simulink model "control_model_flight"  (R2025b)
settings: Solver=VariableStepAuto  StartTime=0.0  StopTime=100  RelTol=1e-3
undefined symbols (not defined in the file): Am, B, Bm, Cm, Dm, engine_gimbal_speed, engine_max_angle, gain, Iy, kd, kp, Kr, Kx, P, static_margin, thrust
libraries: simulink_extras x6, simulink x2
settings Model: Creator=marti  LastModifiedBy=marti
settings DebuggingCC: AlgebraicLoopMsg=none

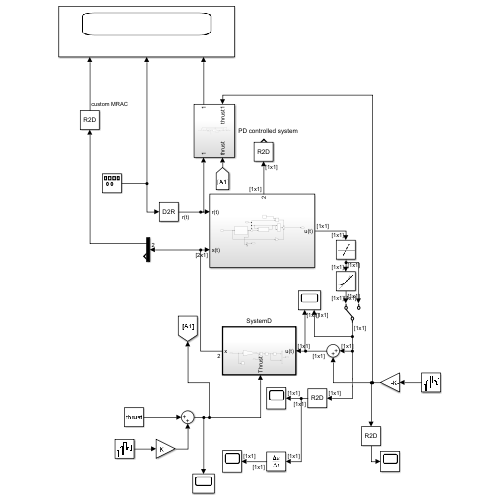
[thumbnail: Simulink's stored preview of the top-level diagram]
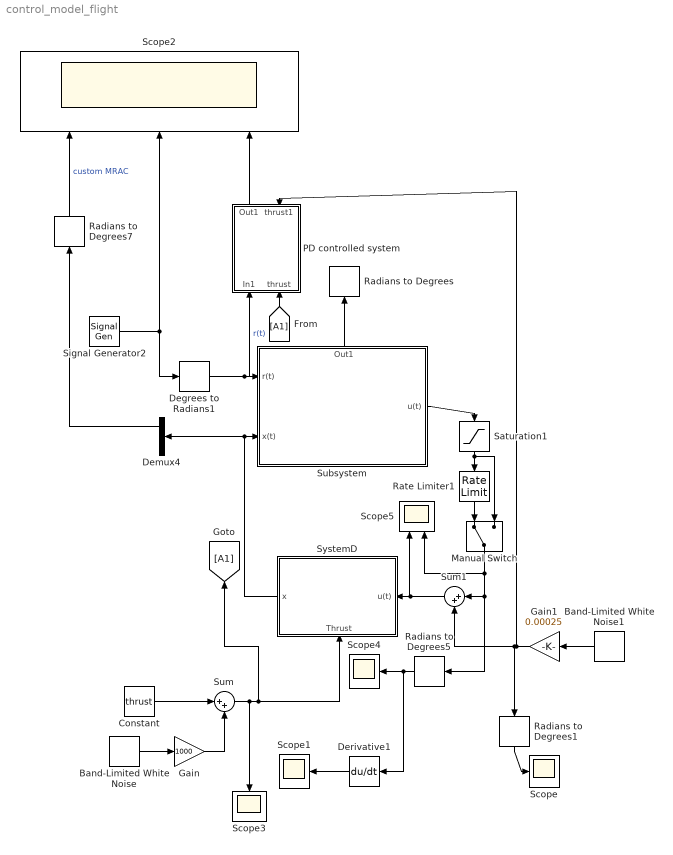
== system control_model_flight ==
  Band-Limited White Noise : simulink/Sources/Band-Limited White Noise  Cov=[0.1]  Ts=1  seed=[23341]
  Band-Limited White Noise1 : simulink/Sources/Band-Limited White Noise  Cov=[0.1]  Ts=0.001  seed=[23341]
  Constant : Constant  Value=thrust
  Degrees to Radians1 : simulink_extras/Transformations/Degrees to Radians
  Demux4 : Demux  Outputs=2
  Derivative1 : Derivative
  Gain : Gain  Gain=1000
  Gain1 : Gain  Gain=0.00025
  Manual Switch : ManualSwitch
  PD controlled system : Subsystem
      settings: PortSchema="{\"entries\":[{\"content\":{\"sides\":[{\"content\":{\"connectorIds\":[\"In1\",\"In2\"]},\"type\":\"ConnectorPlacement.EquallySpacedRectSide\",\"uuid\":\"7664c1e6-ae69-4202-b6ee-140830191e3f\"},{\"content\":{\"connectorIds\":[\"Out1\",\"In3\"],\"side\":\"RIGHT\"},\"type\":\"ConnectorPlacement.EquallySpacedRectSide\",\"uuid\":\"1121b3c6-b64f-4e76-a835-89366e6f1ec3\"},{\"content\":{\"side\":\"TOP\"},\"type\":\"ConnectorPlacement.EquallySpacedRectSide\",\"uuid\":\"4ddc513e-e9d6-44c8-bfb2-5693fffff535\"}]},\"type\":\"ConnectorPlacement.EquallySpacedConnector\",\"uuid\":\"71a54abf-714a-487a-b5bb-d5de61026c0f\"}],\"packageUris\":[\"http://schema.mathworks.com/mf0/Connector/R2020b\"],\"version\":\"1.0\"}"
  Radians to Degrees{,1,5,7} (4 alike) : simulink_extras/Transformations/Radians to Degrees
  Rate Limiter1 : RateLimiter  RisingSlewLimit=engine_gimbal_speed  FallingSlewLimit=-engine_gimbal_speed  SampleTimeMode=inherited
  Saturation1 : Saturate  UpperLimit=engine_max_angle  LowerLimit=-engine_max_angle
  Scope{,1,3..4} (4 alike) : Scope
      Scope settings: ActiveDisplayYMinimum=-1  ActiveDisplayYMaximum=1  DataLoggingVariableName=ScopeData5
      Scope1 settings: ActiveDisplayYMinimum=-573.1584067524692  ActiveDisplayYMaximum=598.11711558803631
      Scope3 settings: ActiveDisplayYMinimum=2853.9945725685793  ActiveDisplayYMaximum=9784.9814242267057  DataLoggingVariableName=ScopeData2
      Scope4 settings: ActiveDisplayYMinimum=-1.2243403544692595  ActiveDisplayYMaximum=1.1538491196054432  DataLoggingVariableName=ScopeData6
  Scope2 : Scope  NumInputPorts=3
      settings: ActiveDisplayYMinimum=-13.72739756342172  ActiveDisplayYMaximum=13.473544890132837
  Scope5 : Scope  NumInputPorts=2
      settings: ActiveDisplayYMinimum=-0.037675490371316969  ActiveDisplayYMaximum=0.03519067284933422  DataLoggingVariableName=ScopeData4
  Signal Generator2 : SignalGenerator  WaveForm=square  Amplitude=10  Frequency=0.1
  Subsystem : Subsystem
      settings: PortSchema="{\"entries\":[{\"content\":{\"sides\":[{\"content\":{\"connectorIds\":[\"In1\",\"In2\"]},\"type\":\"ConnectorPlacement.EquallySpacedRectSide\",\"uuid\":\"2a5405b8-f474-466f-9064-f86b75893dd0\"},{\"content\":{\"connectorIds\":[\"Out1\"],\"side\":\"RIGHT\"},\"type\":\"ConnectorPlacement.EquallySpacedRectSide\",\"uuid\":\"ad673661-f4e9-494b-83cc-7452eec3fe31\"},{\"content\":{\"connectorIds\":[\"Out2\"],\"side\":\"TOP\"},\"type\":\"ConnectorPlacement.EquallySpacedRectSide\",\"uuid\":\"21a76317-3288-4ff3-bd02-68708e86e3a8\"}]},\"type\":\"ConnectorPlacement.EquallySpacedConnector\",\"uuid\":\"fc0ce599-928f-4c66-9629-0b98f2391e21\"}],\"packageUris\":[\"http://schema.mathworks.com/mf0/Connector/R2020b\"],\"version\":\"1.0\"}"
  Sum : Sum  Inputs=|++
  Sum1 : Sum  Inputs=|++
  SystemD : Subsystem  TreatAsAtomicUnit=on
      settings: PortSchema="{\"entries\":[{\"content\":{\"sides\":[{\"content\":{\"connectorIds\":[\"In1\"]},\"type\":\"ConnectorPlacement.EquallySpacedRectSide\",\"uuid\":\"415d6c1e-0406-44b6-8f03-527b0a76a61e\"},{\"content\":{\"connectorIds\":[\"Out1\"],\"side\":\"RIGHT\"},\"type\":\"ConnectorPlacement.EquallySpacedRectSide\",\"uuid\":\"b01fbc7c-daf4-44fd-95a1-f9877c50f20d\"},{\"content\":{\"side\":\"TOP\"},\"type\":\"ConnectorPlacement.EquallySpacedRectSide\",\"uuid\":\"e1a1a26b-9f2a-40fe-9b8c-ace0723ba536\"},{\"content\":{\"connectorIds\":[\"In2\"],\"side\":\"BOTTOM\"},\"type\":\"ConnectorPlacement.EquallySpacedRectSide\",\"uuid\":\"cf849160-1adc-4083-9ccd-983d7a4d3225\"}]},\"type\":\"ConnectorPlacement.EquallySpacedConnector\",\"uuid\":\"7eec5b83-7b07-4bf0-a831-3aced5ecc844\"}],\"packageUris\":[\"http://schema.mathworks.com/mf0/Connector/R2020b\"],\"version\":\"1.0\"}"
  wires:
  Degrees to Radians1/1 -> PD controlled system/1(In1), Subsystem/1(r(t))  "r(t)"
  Saturation1/1 -> Manual Switch/2, Rate Limiter1/1
  Radians to Degrees5/1 -> Derivative1/1, Scope4/1
  Radians to Degrees7/1 -> Scope2/1  "custom MRAC"
  Demux4/1 -> Radians to Degrees7/1
  Derivative1/1 -> Scope1/1
  SystemD/1(x) -> Demux4/1, Subsystem/2(x(t))
  Subsystem/2(Out1) -> Radians to Degrees/1
  PD controlled system/1(Out1) -> Scope2/3
  Signal Generator2/1 -> Degrees to Radians1/1, Scope2/2
  [A1] -> PD controlled system/2(thrust)
  Constant/1 -> Sum/1
  Gain/1 -> Sum/2
  Band-Limited White Noise/1 -> Gain/1
  Sum/1 -> SystemD/2(Thrust), [A1], Scope3/1
  Subsystem/1(u(t)) -> Saturation1/1
  Rate Limiter1/1 -> Manual Switch/1
  Band-Limited White Noise1/1 -> Gain1/1
  Sum1/1 -> Scope5/1, SystemD/1(u(t))
  Gain1/1 -> Radians to Degrees1/1, Sum1/2, PD controlled system/3(thrust1)
  Manual Switch/1 -> Scope5/2, Sum1/1, Radians to Degrees5/1
  Radians to Degrees1/1 -> Scope/1

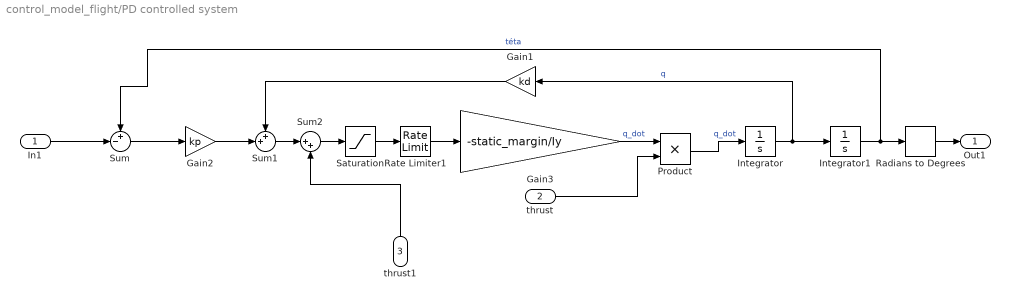
== system control_model_flight/PD controlled system ==
  In1 : Inport
  thrust : Inport  Port=2
  thrust1 : Inport  Port=3
  Gain1 : Gain  Gain=kd
  Gain2 : Gain  Gain=kp
  Gain3 : Gain  Gain=-static_margin/Iy
  Integrator : Integrator
  Integrator1 : Integrator
  Product : Product
  Radians to Degrees : simulink_extras/Transformations/Radians to Degrees
  Rate Limiter1 : RateLimiter  RisingSlewLimit=engine_gimbal_speed  FallingSlewLimit=-engine_gimbal_speed  SampleTimeMode=inherited
  Saturation : Saturate  UpperLimit=engine_max_angle  LowerLimit=-engine_max_angle
  Sum : Sum  Inputs=+-|
  Sum1 : Sum  Inputs=++|
  Sum2 : Sum  Inputs=|++
  Out1 : Outport
  wires:
  Integrator/1 -> Gain1/1, Integrator1/1  "q"
  Gain3/1 -> Product/1  "q_dot"
  thrust/1 -> Product/2
  Gain2/1 -> Sum1/2
  Product/1 -> Integrator/1  "q_dot"
  Gain1/1 -> Sum1/1
  Integrator1/1 -> Radians to Degrees/1, Sum/1  "téta"
  Sum/1 -> Gain2/1
  In1/1 -> Sum/2
  Radians to Degrees/1 -> Out1/1
  Sum1/1 -> Sum2/1
  Sum2/1 -> Saturation/1
  thrust1/1 -> Sum2/2
  Saturation/1 -> Rate Limiter1/1
  Rate Limiter1/1 -> Gain3/1

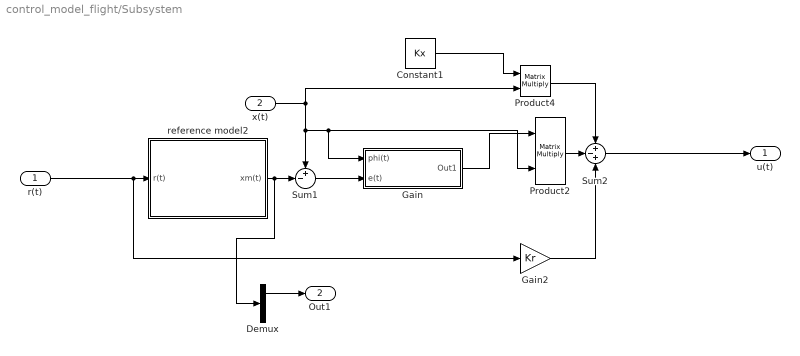
== system control_model_flight/Subsystem ==
  r(t) : Inport
  x(t) : Inport  Port=2  PortDimensions=[2 1]
  Constant1 : Constant  Value=Kx  VectorParams1D=off
  Demux : Demux  Outputs=2
  Gain : Subsystem
  Gain2 : Gain  Gain=Kr
  Product2 : Product  Multiplication=Matrix(*)
  Product4 : Product  Multiplication=Matrix(*)
  Sum1 : Sum  Inputs=+-|
  Sum2 : Sum  Inputs=+-+
  reference model2 : Subsystem  TreatAsAtomicUnit=on
  u(t) : Outport
  Out1 : Outport  Port=2
  wires:
  r(t)/1 -> Gain2/1, reference model2/1(r(t))
  reference model2/1(xm(t)) -> Demux/1, Sum1/2
  x(t)/1 -> Product4/2, Product2/2, Gain/1(phi(t)), Sum1/1
  Product2/1 -> Sum2/2
  Sum1/1 -> Gain/2(e(t))
  Constant1/1 -> Product4/1
  Product4/1 -> Sum2/1
  Gain2/1 -> Sum2/3
  Sum2/1 -> u(t)/1
  Gain/1(Out1) -> Product2/1
  Demux/1 -> Out1/1

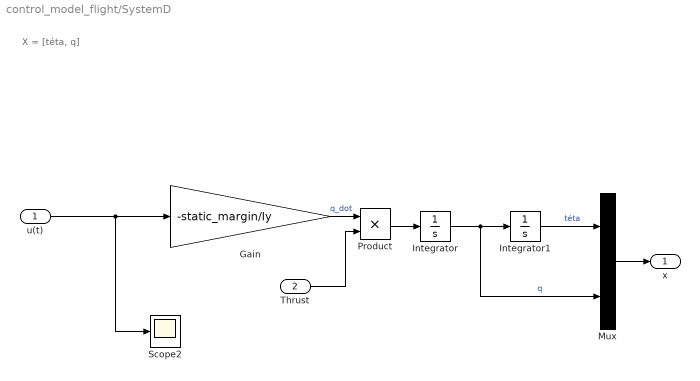
== system control_model_flight/SystemD ==
  note: X = [téta, q]
  u(t) : Inport
  Thrust : Inport  Port=2
  Gain : Gain  Gain=-static_margin/Iy
  Integrator : Integrator
  Integrator1 : Integrator
  Mux : Mux  Inputs=2
  Product : Product
  Scope2 : Scope
      settings: ActiveDisplayYMinimum=-1  ActiveDisplayYMaximum=1  DataLoggingVariableName=ScopeData3
  x : Outport
  wires:
  Integrator/1 -> Integrator1/1, Mux/2  "q"
  Integrator1/1 -> Mux/1  "téta"
  Mux/1 -> x/1
  u(t)/1 -> Scope2/1, Gain/1
  Gain/1 -> Product/1  "q_dot"
  Product/1 -> Integrator/1
  Thrust/1 -> Product/2

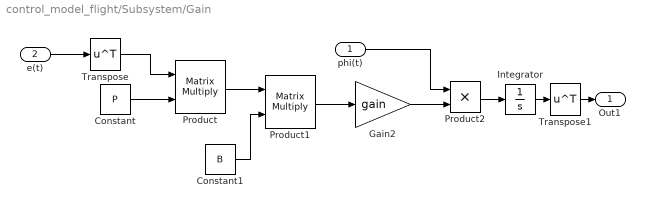
== system control_model_flight/Subsystem/Gain ==
  phi(t) : Inport
  e(t) : Inport  Port=2
  Constant : Constant  Value=P  VectorParams1D=off
  Constant1 : Constant  Value=B  VectorParams1D=off
  Gain2 : Gain  Gain=gain
  Integrator : Integrator
  Product : Product  Multiplication=Matrix(*)
  Product1 : Product  Multiplication=Matrix(*)
  Product2 : Product
  Transpose : Math  Operator=transpose
  Transpose1 : Math  Operator=transpose
  Out1 : Outport
  wires:
  Product1/1 -> Gain2/1
  phi(t)/1 -> Product2/1
  Product/1 -> Product1/1
  Constant1/1 -> Product1/2
  Gain2/1 -> Product2/2
  e(t)/1 -> Transpose/1
  Constant/1 -> Product/2
  Transpose/1 -> Product/1
  Product2/1 -> Integrator/1
  Integrator/1 -> Transpose1/1
  Transpose1/1 -> Out1/1

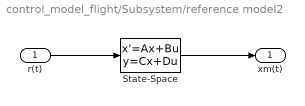
== system control_model_flight/Subsystem/reference model2 ==
  r(t) : Inport
  State-Space : StateSpace  A=Am  B=Bm  C=Cm  D=Dm  InitialCondition=[0;0]
  xm(t) : Outport  PortDimensions=[2 1]
  wires:
  State-Space/1 -> xm(t)/1
  r(t)/1 -> State-Space/1
